simulink model "withPattern"  (R2020a)
settings: Solver=VariableStepAuto  StartTime=0.0  StopTime=0.5  RelTol=1e-3
model workspace (MAT data in the model file):
  Ts = 0.1
libraries: simulink x1
settings Model: Creator=liuzhenjie  LastModifiedBy=liuzhenjie

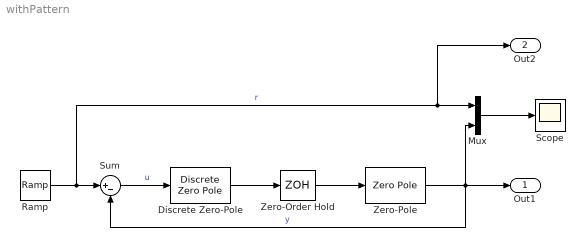
== system withPattern ==
  Discrete Zero-Pole : DiscreteZeroPole  Zeros=|  Poles=|  Gain=82.6887  SampleTime=Ts
      Zeros=|
      | [ 0.5000
      |     0.9048]
      Poles=|
      | [   -0.9672
      |     1.0000]
  Mux : Mux  Inputs=2
  Ramp : simulink/Sources/Ramp  slope=1  start=0  InitialOutput=0
  Scope : Scope
  Sum : Sum  Inputs=|+-
  Zero-Order Hold : ZeroOrderHold  SampleTime=Ts
  Zero-Pole : ZeroPole  Zeros=[]  Poles=[0 -1]  Gain=5
  Out1 : Outport
  Out2 : Outport  Port=2
  wires:
  Ramp/1 -> Out2/1, Mux/1, Sum/1  "r"
  Sum/1 -> Discrete Zero-Pole/1  "u"
  Discrete Zero-Pole/1 -> Zero-Order Hold/1
  Zero-Order Hold/1 -> Zero-Pole/1
  Zero-Pole/1 -> Mux/2, Sum/2, Out1/1  "y"
  Mux/1 -> Scope/1
